simulink model "linearizedModel"  (R2022b)
settings: Solver=VariableStepAuto  StartTime=0.0  StopTime=100  RelTol=1e-3
values from neighbouring files (symbols this model uses):
  A = zeros(6,6)    [sim1_PartD.m]    (also in sim2_PartF.m; sim3_partG_part1.m; sim4_partG_part2.m)
  B = [0,1/M,0,-1/M/l1,0,-1/M/l2]'    [sim1_PartD.m]    (also in sim2_PartF.m)
  C = zeros(3,6)    [sim1_PartD.m]    (also in sim2_PartF.m = [1,0,0,0,0,0; sim3_partG_part1.m = CC(var_sel,:); sim4_partG_part2.m = CC(var_sel,:))
  D = zeros(3,1)    [sim1_PartD.m]    (also in sim2_PartF.m = zeros(size(C,1),1); sim3_partG_part1.m = zeros(n_output_var,1); sim4_partG_part2.m = zeros(n_output_var,1))
  init_state = [x0,xd0,theta1_0,theta1_d0,theta2_0,theta2_d0]'    [sim1_PartD.m]    (also in sim2_PartF.m = [5,-0.5,20/180*pi,-0.5,-20/180*pi,0.5]'; sim3_partG_part1.m = [5,-0.5,20/180*pi,-0.5,-20/180*pi,0.5]'; sim4_partG_part2.m = [0,0,0,0,0,0]')
  K = -K    [sim1_PartD.m]    (also in sim3_partG_part1.m)
settings Model: Creator=liuji  LastModifiedBy=liuji

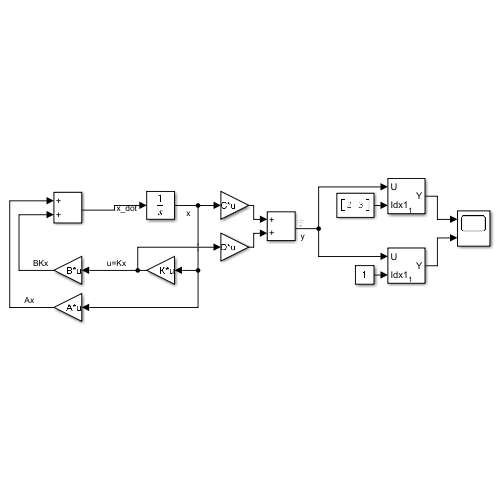
[thumbnail: Simulink's stored preview of the top-level diagram]
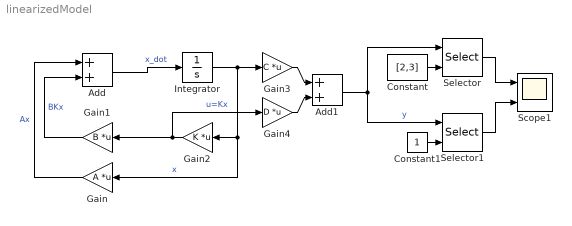
== system linearizedModel ==
  Add : Sum
  Add1 : Sum
  Constant : Constant  Value=[2,3]
  Constant1 : Constant
  Gain : Gain  Gain=A  Multiplication=Matrix(K*u)
  Gain1 : Gain  Gain=B  Multiplication=Matrix(K*u)
  Gain2 : Gain  Gain=K  Multiplication=Matrix(K*u)
  Gain3 : Gain  Gain=C  Multiplication=Matrix(K*u)
  Gain4 : Gain  Gain=D  Multiplication=Matrix(K*u)
  Integrator : Integrator  InitialCondition=init_state
  Scope1 : Scope  NumInputPorts=2
  Selector : Selector  InputPortWidth=3  IndexOptions=Index vector (port)  Indices=[1 3]  OutputSizes=1
  Selector1 : Selector  InputPortWidth=3  IndexOptions=Index vector (port)  Indices=[1 3]  OutputSizes=1
  wires:
  Integrator/1 -> Gain3/1, Gain/1, Gain2/1  "x"
  Gain2/1 -> Gain1/1, Gain4/1  "u=Kx"
  Add/1 -> Integrator/1  "x_dot"
  Gain/1 -> Add/1  "Ax"
  Gain3/1 -> Add1/1
  Gain4/1 -> Add1/2
  Add1/1 -> Selector1/1, Selector/1  "y"
  Constant/1 -> Selector/2
  Selector/1 -> Scope1/1
  Constant1/1 -> Selector1/2
  Selector1/1 -> Scope1/2
  Gain1/1 -> Add/2  "BKx"
